simulink model "part_3_2"  (R2025a)
settings: Solver=FixedStepAuto  StartTime=0.0  StopTime=400  FixedStep=0.0005  RelTol=1e-3
values from neighbouring files (symbols this model uses):
  kts_to_ms = 0.5144444444    [constants.m]
  q0 = 0    [part_3_2_params.m]
  theta_f_0 = atan2(-D0,p.W)    [part_3_2_params.m]
  u0 = V0 * cos(theta_f_0)    [part_3_2_params.m]
  w0 = V0 * sin(theta_f_0)    [part_3_2_params.m]
undefined symbols (not defined in the file or in its folder): theta_0_trim
libraries: slpidlib x3, simulink x1
settings Model: Creator=niels  LastModifiedBy=niels

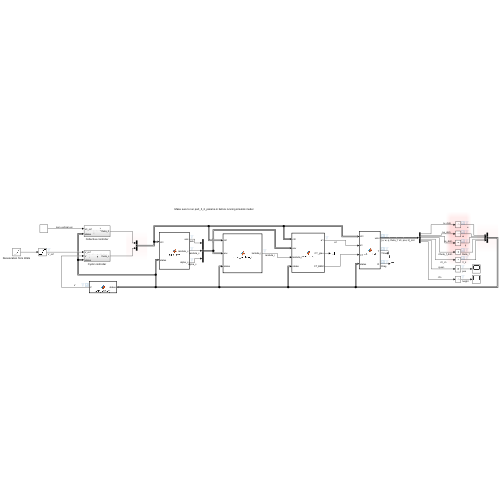
[thumbnail: Simulink's stored preview of the top-level diagram]
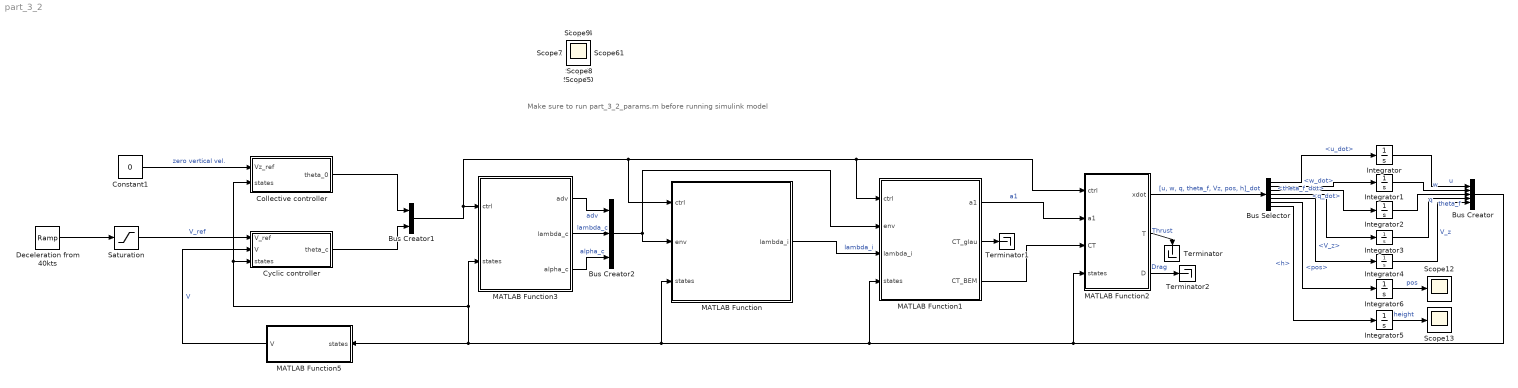
== system part_3_2 ==
  note: Make sure to run part_3_2_params.m before running simulink model
  Bus Creator : BusCreator  Inputs=5  OutDataTypeStr=Bus: slBus1
  Bus Creator1 : BusCreator  Inputs=2  OutDataTypeStr=Bus: slBus2
  Bus Creator2 : BusCreator  Inputs=3
  Bus Selector : BusSelector  OutputSignals=u_dot,w_dot,q_dot,theta_f_dot,V_z,pos,h
  Collective controller : Subsystem
  Constant1 : Constant  Value=0
  Cyclic controller : Subsystem
  Deceleration from 40kts : simulink/Sources/Ramp  slope=-1 * kts_to_ms  start=5  InitialOutput=40 * kts_to_ms
  Integrator : Integrator  InitialCondition=u0
  Integrator1 : Integrator  InitialCondition=w0
  Integrator2 : Integrator  InitialCondition=q0
  Integrator3 : Integrator  InitialCondition=theta_f_0
  Integrator4 : Integrator
  Integrator5 : Integrator
  Integrator6 : Integrator
  MATLAB Function : MATLAB Function  TreatAsAtomicUnit=on
  MATLAB Function1 : MATLAB Function  TreatAsAtomicUnit=on
  MATLAB Function2 : MATLAB Function  TreatAsAtomicUnit=on
  MATLAB Function3 : MATLAB Function  TreatAsAtomicUnit=on
  MATLAB Function5 : MATLAB Function  TreatAsAtomicUnit=on
  Saturation : Saturate  UpperLimit=40 * kts_to_ms  LowerLimit=0
  Scope{,1..13} (14 alike) : Scope
      Scope12 settings: ActiveDisplayYMinimum=-66.519454553298687  ActiveDisplayYMaximum=598.67509097968832  DataLoggingVariableName=ScopeData12
      Scope13 settings: ActiveDisplayYMinimum=-0.8759795141479535  ActiveDisplayYMaximum=0.71117795186084842  DataLoggingVariableName=ScopeData13
      Scope settings: ActiveDisplayYMinimum=-69.673258872485547  ActiveDisplayYMaximum=96.001341434570236
      Scope1 settings: ActiveDisplayYMinimum=-4.975868665333758  ActiveDisplayYMaximum=4.3203867980241615
      Scope10 settings: ActiveDisplayYMinimum=-1  ActiveDisplayYMaximum=1  DataLoggingVariableName=ScopeData10
      Scope11 settings: ActiveDisplayYMinimum=-0.16112339475038778  ActiveDisplayYMaximum=0.36190773098455026  DataLoggingVariableName=ScopeData11
      Scope2 settings: ActiveDisplayYMinimum=-0.593397020253839  ActiveDisplayYMaximum=52.786649391478015  DataLoggingVariableName=ScopeData2
      Scope3 settings: ActiveDisplayYMinimum=-78.6156985163187  ActiveDisplayYMaximum=71.050366553263416  DataLoggingVariableName=ScopeData3
      Scope4 settings: ActiveDisplayYMinimum=-4497.44134433289  ActiveDisplayYMaximum=2027.1404146909797  DataLoggingVariableName=ScopeData4
      Scope5 settings: ActiveDisplayYMinimum=-24353.236413473656  ActiveDisplayYMaximum=7406.41209327752  DataLoggingVariableName=ScopeData5
      Scope6 settings: DataLoggingVariableName=ScopeData6
      Scope7 settings: DataLoggingVariableName=ScopeData7
      Scope8 settings: ActiveDisplayYMinimum=-71153.912510590511  ActiveDisplayYMaximum=70611.962806822383  DataLoggingVariableName=ScopeData8
      Scope9 settings: ActiveDisplayYMinimum=-197167.0431723232  ActiveDisplayYMaximum=258208.12713879911  DataLoggingVariableName=ScopeData9
  Terminator : Terminator
  Terminator1 : Terminator
  Terminator2 : Terminator
  wires:
  MATLAB Function3/1(adv) -> Bus Creator2/1  "adv"
  MATLAB Function/1(lambda_i) -> MATLAB Function1/3(lambda_i)  "lambda_i"
  MATLAB Function1/1(a1) -> MATLAB Function2/2(a1)  "a1"
  MATLAB Function5/1(V) -> Cyclic controller/2(V)  "V"
  MATLAB Function1/3(CT_BEM) -> MATLAB Function2/3(CT)
  MATLAB Function3/2(lambda_c) -> Bus Creator2/2  "lambda_c"
  MATLAB Function3/3(alpha_c) -> Bus Creator2/3  "alpha_c"
  Bus Creator1/1 -> MATLAB Function2/1(ctrl), MATLAB Function1/1(ctrl), MATLAB Function/1(ctrl), MATLAB Function3/1(ctrl)
  MATLAB Function2/1(xdot) -> Bus Selector/1  "[u, w, q, theta_f, Vz, pos, h]_dot"
  Bus Selector/1 -> Integrator/1  "<u_dot>"
  Bus Selector/2 -> Integrator1/1  "<w_dot>"
  Integrator/1 -> Bus Creator/1  "u"
  Integrator1/1 -> Bus Creator/2  "w"
  Integrator2/1 -> Bus Creator/3  "q"
  Integrator3/1 -> Bus Creator/4  "theta_f"
  Bus Selector/3 -> Integrator2/1  "<q_dot>"
  Bus Creator/1 -> MATLAB Function2/4(states), MATLAB Function1/4(states), MATLAB Function/3(states), Collective controller/2(states), Cyclic controller/3(states), MATLAB Function3/2(states), MATLAB Function5/1(states)
  MATLAB Function2/2(T) -> Terminator/1  "Thrust"
  MATLAB Function2/3(D) -> Terminator2/1  "Drag"
  Bus Creator2/1 -> MATLAB Function/2(env), MATLAB Function1/2(env)
  Collective controller/1(theta_0) -> Bus Creator1/1
  Cyclic controller/1(theta_c) -> Bus Creator1/2
  Bus Selector/4 -> Integrator3/1  "<theta_f_dot>"
  Constant1/1 -> Collective controller/1(Vz_ref)  "zero vertical vel."
  Bus Selector/5 -> Integrator4/1  "<V_z>"
  Integrator4/1 -> Bus Creator/5  "V_z"
  Saturation/1 -> Cyclic controller/1(V_ref)  "V_ref"
  Deceleration from 40kts/1 -> Saturation/1
  Bus Selector/6 -> Integrator6/1  "<pos>"
  Bus Selector/7 -> Integrator5/1  "<h>"
  Integrator6/1 -> Scope12/1  "pos"
  Integrator5/1 -> Scope13/1  "height"
  MATLAB Function1/2(CT_glau) -> Terminator1/1

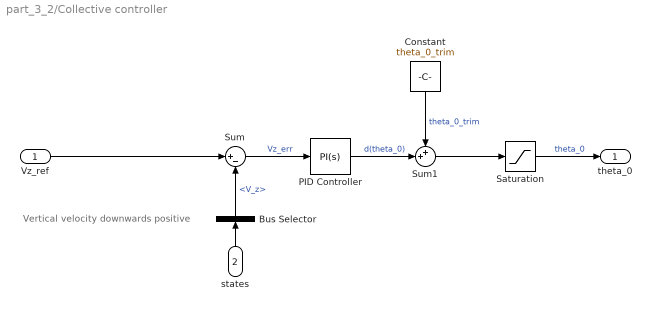
== system part_3_2/Collective controller ==
  note: Vertical velocity downwards positive
  Vz_ref : Inport
  states : Inport  Port=2
  Bus Selector : BusSelector  OutputSignals=V_z
  Constant : Constant  Value=theta_0_trim
  PID Controller : slpidlib/PID Controller  Controller=PI  Form=Parallel  TimeDomain=Continuous-time  UseExternalTs=off  SampleTime=-1  IntegratorMethod=Forward Euler  FilterMethod=Forward Euler  ControllerParametersSource=internal  P=0.356905218737675  I=3.63280538861423  UseKiTs=off  D=0  UseExternalDerivativeSource=off  N=100  UseFilter=on  TunerSelectOption=Transfer Function Based (PID Tuner App)  InitialConditionSource=internal  InitialConditionForIntegrator=0  InitialConditionForFilter=0  DifferentiatorICPrevScaledInput=0  ExternalReset=none  TrackingMode=off  Kt=1  LimitOutput=on  SatLimitsSource=internal  UpperSaturationLimit=inf  LowerSaturationLimit=-inf  LinearizeAsGain=on  AntiWindupMode=back-calculation  Kb=1/1.7722615314585  LimitIntegrator=off  UpperIntegratorSaturationLimit=inf  LowerIntegratorSaturationLimit=-inf  POutMin=[]  POutMax=[]  IOutMin=[]  IOutMax=[]  DOutMin=[]  DOutMax=[]  NOutMin=[]  NOutMax=[]  SumOutMin=[]  SumOutMax=[]  SaturationOutMin=[]  SaturationOutMax=[]  PParamMin=[]  PParamMax=[]  IParamMin=[]  IParamMax=[]  DParamMin=[]  DParamMax=[]  NParamMin=[]  NParamMax=[]  KbParamMin=[]  KbParamMax=[]  KtParamMin=[]  KtParamMax=[]  KbOutMin=[]  KbOutMax=[]  KtOutMin=[]  KtOutMax=[]  IntegratorOutMin=[]  IntegratorOutMax=[]  FilterOutMin=[]  FilterOutMax=[]  SumI1OutMin=[]  SumI1OutMax=[]  SumI2OutMin=[]  SumI2OutMax=[]  SumI3OutMin=[]  SumI3OutMax=[]  SumI4OutMin=[]  SumI4OutMax=[]  SumDOutMin=[]  SumDOutMax=[]  DifferentiatorOutMin=[]  DifferentiatorOutMax=[]  FilterDiffOutCoefMin=[]  FilterDiffOutCoefMax=[]  ReciprocalOutMin=[]  ReciprocalOutMax=[]  SumDenOutMin=[]  SumDenOutMax=[]  SumNumOutMin=[]  SumNumOutMax=[]  DivideOutMin=[]  DivideOutMax=[]  UdiffTsProdOutMin=[]  UdiffTsProdOutMax=[]  NTsProdOutMin=[]  NTsProdOutMax=[]  UintegralTsProdOutMin=[]  UintegralTsProdOutMax=[]  UngainTsProdOutMin=[]  UngainTsProdOutMax=[]  ClampingZeroOutDataTypeStr=Inherit: Inherit via back propagation  ClampingZeroOutMin=[]  ClampingZeroOutMax=[]  FilterDenConstantOutDataTypeStr=Inherit: Inherit via back propagation  FilterDenConstantOutMin=[]  FilterDenConstantOutMax=[]  PCopyOutDataTypeStr=Inherit: Inherit via back propagation  PCopyOutMin=[]  PCopyOutMax=[]  NCopyOutDataTypeStr=Inherit: Inherit via back propagation  NCopyOutMin=[]  NCopyOutMax=[]  IntegratorContinuousStateAttributes=''  IntegratorStateMustResolveToSignalObject=off  IntegratorRTWStateStorageClass=Auto  FilterContinuousStateAttributes=''  FilterStateMustResolveToSignalObject=off  FilterRTWStateStorageClass=Auto  ParallelPVariant=InternalParameters  IdealPVariant=Disabled  IVariant=InternalParameters  DVariant=Disabled  IntegratorVariant=Continuous  SatVariant=Enabled  AWVariant=BackCalculation  PCopyVariant=Disabled  TRVariant=Disabled  FdbkBlocksVariant=Forward  IdealPFdbkVariant=Disabled  SatFdbkVariant=Disabled  DerivativeFilterVariant=Disabled  NVariant=Disabled  NCopyVariant=Disabled_SignalSpec  FilterICVariant=Disabled  IntegratorICVariant=InternalICs  ExternalResetVariant=Disabled  TRSumVariant=Passthrough  SumFdbkVariant=Disabled  SumVariant=Sum_PI  TsampFilterVariant=InternalTs  TsampNgainVariant=Passthrough  TsampIntegralVariant=Disabled_SignalSpec  ExternalSaturationOutDataTypeStr=Inherit: Same as second input  DerivativeSourceVariant=Disabled  PreIntVariant=InternalPreInt
  Saturation : Saturate  UpperLimit=22.7*pi/180  LowerLimit=4*pi/180  LinearizeAsGain=off
  Sum : Sum  Inputs=|+-
  Sum1 : Sum  Inputs=++|
  theta_0 : Outport
  wires:
  Vz_ref/1 -> Sum/1
  Constant/1 -> Sum1/1  "theta_0_trim"
  Sum1/1 -> Saturation/1
  Sum/1 -> PID Controller/1  "Vz_err"
  PID Controller/1 -> Sum1/2  "d(theta_0)"
  Saturation/1 -> theta_0/1  "theta_0"
  states/1 -> Bus Selector/1
  Bus Selector/1 -> Sum/2  "<V_z>"

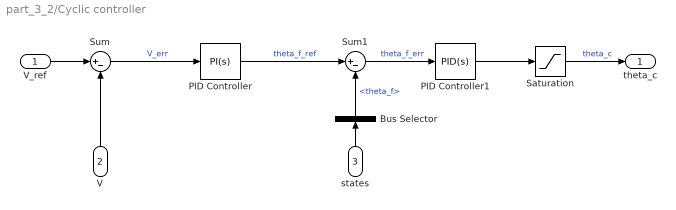
== system part_3_2/Cyclic controller ==
  V_ref : Inport
  V : Inport  Port=2
  states : Inport  Port=3
  Bus Selector : BusSelector  OutputSignals=theta_f
  PID Controller : slpidlib/PID Controller  Controller=PI  Form=Parallel  TimeDomain=Continuous-time  UseExternalTs=off  SampleTime=-1  IntegratorMethod=Forward Euler  FilterMethod=Forward Euler  ControllerParametersSource=internal  P=-0.0818787795811215  I=-0.000899384749307426  UseKiTs=off  D=0  UseExternalDerivativeSource=off  N=100  UseFilter=on  TunerSelectOption=Transfer Function Based (PID Tuner App)  InitialConditionSource=internal  InitialConditionForIntegrator=0  InitialConditionForFilter=0  DifferentiatorICPrevScaledInput=0  ExternalReset=none  TrackingMode=off  Kt=1  LimitOutput=off  SatLimitsSource=internal  UpperSaturationLimit=inf  LowerSaturationLimit=-inf  LinearizeAsGain=on  AntiWindupMode=none  Kb=1  LimitIntegrator=off  UpperIntegratorSaturationLimit=inf  LowerIntegratorSaturationLimit=-inf  POutMin=[]  POutMax=[]  IOutMin=[]  IOutMax=[]  DOutMin=[]  DOutMax=[]  NOutMin=[]  NOutMax=[]  SumOutMin=[]  SumOutMax=[]  SaturationOutMin=[]  SaturationOutMax=[]  PParamMin=[]  PParamMax=[]  IParamMin=[]  IParamMax=[]  DParamMin=[]  DParamMax=[]  NParamMin=[]  NParamMax=[]  KbParamMin=[]  KbParamMax=[]  KtParamMin=[]  KtParamMax=[]  KbOutMin=[]  KbOutMax=[]  KtOutMin=[]  KtOutMax=[]  IntegratorOutMin=[]  IntegratorOutMax=[]  FilterOutMin=[]  FilterOutMax=[]  SumI1OutMin=[]  SumI1OutMax=[]  SumI2OutMin=[]  SumI2OutMax=[]  SumI3OutMin=[]  SumI3OutMax=[]  SumI4OutMin=[]  SumI4OutMax=[]  SumDOutMin=[]  SumDOutMax=[]  DifferentiatorOutMin=[]  DifferentiatorOutMax=[]  FilterDiffOutCoefMin=[]  FilterDiffOutCoefMax=[]  ReciprocalOutMin=[]  ReciprocalOutMax=[]  SumDenOutMin=[]  SumDenOutMax=[]  SumNumOutMin=[]  SumNumOutMax=[]  DivideOutMin=[]  DivideOutMax=[]  UdiffTsProdOutMin=[]  UdiffTsProdOutMax=[]  NTsProdOutMin=[]  NTsProdOutMax=[]  UintegralTsProdOutMin=[]  UintegralTsProdOutMax=[]  UngainTsProdOutMin=[]  UngainTsProdOutMax=[]  ClampingZeroOutDataTypeStr=Inherit: Inherit via back propagation  ClampingZeroOutMin=[]  ClampingZeroOutMax=[]  FilterDenConstantOutDataTypeStr=Inherit: Inherit via back propagation  FilterDenConstantOutMin=[]  FilterDenConstantOutMax=[]  PCopyOutDataTypeStr=Inherit: Inherit via back propagation  PCopyOutMin=[]  PCopyOutMax=[]  NCopyOutDataTypeStr=Inherit: Inherit via back propagation  NCopyOutMin=[]  NCopyOutMax=[]  IntegratorContinuousStateAttributes=''  IntegratorStateMustResolveToSignalObject=off  IntegratorRTWStateStorageClass=Auto  FilterContinuousStateAttributes=''  FilterStateMustResolveToSignalObject=off  FilterRTWStateStorageClass=Auto  ParallelPVariant=InternalParameters  IdealPVariant=Disabled  IVariant=InternalParameters  DVariant=Disabled  IntegratorVariant=Continuous  SatVariant=Disabled  AWVariant=Passthrough  PCopyVariant=Disabled  TRVariant=Disabled  FdbkBlocksVariant=Forward  IdealPFdbkVariant=Disabled  SatFdbkVariant=Disabled  DerivativeFilterVariant=Disabled  NVariant=Disabled  NCopyVariant=Disabled_SignalSpec  FilterICVariant=Disabled  IntegratorICVariant=InternalICs  ExternalResetVariant=Disabled  TRSumVariant=Passthrough  SumFdbkVariant=Disabled  SumVariant=Sum_PI  TsampFilterVariant=InternalTs  TsampNgainVariant=Passthrough  TsampIntegralVariant=Disabled_SignalSpec  ExternalSaturationOutDataTypeStr=Inherit: Same as second input  DerivativeSourceVariant=Disabled  PreIntVariant=InternalPreInt
  PID Controller1 : slpidlib/PID Controller  Controller=PID  Form=Parallel  TimeDomain=Continuous-time  UseExternalTs=off  SampleTime=-1  IntegratorMethod=Forward Euler  FilterMethod=Forward Euler  ControllerParametersSource=internal  P=-74.2488008539596  I=-94.6679783127372  UseKiTs=off  D=-14.3024383116871  UseExternalDerivativeSource=off  N=147.428825111733  UseFilter=on  TunerSelectOption=Transfer Function Based (PID Tuner App)  InitialConditionSource=internal  InitialConditionForIntegrator=0  InitialConditionForFilter=0  DifferentiatorICPrevScaledInput=0  ExternalReset=none  TrackingMode=off  Kt=1  LimitOutput=off  SatLimitsSource=internal  UpperSaturationLimit=inf  LowerSaturationLimit=-inf  LinearizeAsGain=on  AntiWindupMode=back-calculation  Kb=1/22.8221920607983  LimitIntegrator=off  UpperIntegratorSaturationLimit=inf  LowerIntegratorSaturationLimit=-inf  POutMin=[]  POutMax=[]  IOutMin=[]  IOutMax=[]  DOutMin=[]  DOutMax=[]  NOutMin=[]  NOutMax=[]  SumOutMin=[]  SumOutMax=[]  SaturationOutMin=[]  SaturationOutMax=[]  PParamMin=[]  PParamMax=[]  IParamMin=[]  IParamMax=[]  DParamMin=[]  DParamMax=[]  NParamMin=[]  NParamMax=[]  KbParamMin=[]  KbParamMax=[]  KtParamMin=[]  KtParamMax=[]  KbOutMin=[]  KbOutMax=[]  KtOutMin=[]  KtOutMax=[]  IntegratorOutMin=[]  IntegratorOutMax=[]  FilterOutMin=[]  FilterOutMax=[]  SumI1OutMin=[]  SumI1OutMax=[]  SumI2OutMin=[]  SumI2OutMax=[]  SumI3OutMin=[]  SumI3OutMax=[]  SumI4OutMin=[]  SumI4OutMax=[]  SumDOutMin=[]  SumDOutMax=[]  DifferentiatorOutMin=[]  DifferentiatorOutMax=[]  FilterDiffOutCoefMin=[]  FilterDiffOutCoefMax=[]  ReciprocalOutMin=[]  ReciprocalOutMax=[]  SumDenOutMin=[]  SumDenOutMax=[]  SumNumOutMin=[]  SumNumOutMax=[]  DivideOutMin=[]  DivideOutMax=[]  UdiffTsProdOutMin=[]  UdiffTsProdOutMax=[]  NTsProdOutMin=[]  NTsProdOutMax=[]  UintegralTsProdOutMin=[]  UintegralTsProdOutMax=[]  UngainTsProdOutMin=[]  UngainTsProdOutMax=[]  ClampingZeroOutDataTypeStr=Inherit: Inherit via back propagation  ClampingZeroOutMin=[]  ClampingZeroOutMax=[]  FilterDenConstantOutDataTypeStr=Inherit: Inherit via back propagation  FilterDenConstantOutMin=[]  FilterDenConstantOutMax=[]  PCopyOutDataTypeStr=Inherit: Inherit via back propagation  PCopyOutMin=[]  PCopyOutMax=[]  NCopyOutDataTypeStr=Inherit: Inherit via back propagation  NCopyOutMin=[]  NCopyOutMax=[]  IntegratorContinuousStateAttributes=''  IntegratorStateMustResolveToSignalObject=off  IntegratorRTWStateStorageClass=Auto  FilterContinuousStateAttributes=''  FilterStateMustResolveToSignalObject=off  FilterRTWStateStorageClass=Auto  ParallelPVariant=InternalParameters  IdealPVariant=Disabled  IVariant=InternalParameters  DVariant=InternalParameters  IntegratorVariant=Continuous  SatVariant=Disabled  AWVariant=Passthrough  PCopyVariant=Disabled  TRVariant=Disabled  FdbkBlocksVariant=Forward  IdealPFdbkVariant=Disabled  SatFdbkVariant=Disabled  DerivativeFilterVariant=ContFilter  NVariant=InternalParameters  NCopyVariant=Disabled  FilterICVariant=InternalICsFilter  IntegratorICVariant=InternalICs  ExternalResetVariant=Disabled  TRSumVariant=Passthrough  SumFdbkVariant=Disabled  SumVariant=Sum_PID  TsampFilterVariant=InternalTs  TsampNgainVariant=Passthrough  TsampIntegralVariant=Disabled_SignalSpec  ExternalSaturationOutDataTypeStr=Inherit: Same as second input  DerivativeSourceVariant=ErrorSignal  PreIntVariant=InternalPreInt
  Saturation : Saturate  UpperLimit=19.25*pi/180  LowerLimit=-14.75*pi/180
  Sum : Sum  Inputs=|+-
  Sum1 : Sum  Inputs=|+-
  theta_c : Outport
  wires:
  V_ref/1 -> Sum/1
  V/1 -> Sum/2
  Sum/1 -> PID Controller/1  "V_err"
  Sum1/1 -> PID Controller1/1  "theta_f_err"
  PID Controller1/1 -> Saturation/1
  Saturation/1 -> theta_c/1  "theta_c"
  PID Controller/1 -> Sum1/1  "theta_f_ref"
  states/1 -> Bus Selector/1
  Bus Selector/1 -> Sum1/2  "<theta_f>"

== matlab function part_3_2/MATLAB Function1 ==
  data: ctrl input Bus: slBus2; env input Bus: slBus4; lambda_i input; a1 output; CT_glau output; states input Bus: slBus1; CT_BEM output; p parameter
function [a1, CT_glau, CT_BEM] = ...
            calc_aero(ctrl, env, lambda_i, states, p)

    theta_0 = ctrl.theta_0;
    q = states.q;
    adv = env.adv;
    lambda_c = env.lambda_c;
    alpha_c = env.alpha_c;
    
    % a1: longitudinal flapping angle
    num   = (8/3)*adv*theta_0 - 2*adv*(lambda_c + lambda_i) ...
                - (16/p.Lock)*(q/p.OmegaR);
    den = 1 - 0.5*adv^2;
    if abs(den) < 1e-8
        den = sign(den + eps) * 1e-8;
    end
    
    a1 = num / den;

    % CT_BEM: Blade Element Momentum thrust coefficient
    CT_BEM = p.cl_alpha * (1/4) * (p.sigma) * ((2/3)*theta_0* ...
                (1 + (3/2)*adv^2) - (lambda_c + lambda_i));

    % CT_glau: Glauert thrust coefficient
    Vc_norm = adv * cos(alpha_c - a1);
    Vs_norm = adv * sin(alpha_c - a1);

    CT_glau = 2 * lambda_i * sqrt( Vc_norm^2 + (Vs_norm + lambda_i)^2 );

end

== matlab function part_3_2/MATLAB Function ==
  data: ctrl input Bus: slBus2; env input Bus: slBus4; lambda_i output; states input Bus: slBus1; p parameter
function lambda_i  = ...
            solve_lambda_i(ctrl, env, states, p)
% Solves for lambda_i such that F(lambda_i) = C_TBEM - C_TGlau = 0
%
% Inputs:
%   adv      - advance ratio [-]
%   theta_0  - collective pitch [rad]
%   lambda_c - climb inflow ratio
%   q        - some loading parameter
%   alpha_c  - shaft/disc tilt angle [rad]
%   p        - data struct
    theta_0 = ctrl.theta_0;
    q = states.q;
    adv = env.adv;
    lambda_c = env.lambda_c;
    alpha_c = env.alpha_c;

    % Define the residual function F(lambda_i) = C_TBEM - C_TGlau
    F = @(lambda_i) residual(lambda_i, adv, theta_0, lambda_c, q, ...
                                alpha_c, p);

    % Initial guess for lambda_i
    lambda_i0 = 0.05;

    % Solve using fzero
    lambda_i = fzero(F, lambda_i0);

    fprintf('Converged: lambda_i = %.6f\n', lambda_i);
end

function F = residual(lambda_i, adv, theta_0, lambda_c, q, alpha_c, p)

    % a1: longitudinal flapping angle
    num   = (8/3)*adv*theta_0 - 2*adv*(lambda_c + lambda_i) ...
                - (16/p.Lock)*(q/p.OmegaR);
    den = 1 - 0.5*adv^2;
    if abs(den) < 1e-8
        den = sign(den + eps) * 1e-8;
    end
    
    a1 = num / den;

    % CT_BEM: Blade Element Momentum thrust coefficient
    CT_BEM = p.cl_alpha * (1/4) * (p.sigma) * ((2/3)*theta_0* ...
                (1 + (3/2)*adv^2) - (lambda_c + lambda_i));

    % CT_glau: Glauert thrust coefficient
    Vc_norm = adv * cos(alpha_c - a1);
    Vs_norm = adv * sin(alpha_c - a1);

    CT_glau = 2 * lambda_i * sqrt( Vc_norm^2 + (Vs_norm + lambda_i)^2 );

    % Residual
    F = CT_BEM - CT_glau;
end

== matlab function part_3_2/MATLAB Function2 ==
  data: ctrl input Bus: slBus2; a1 input; CT input; states input Bus: slBus1; xdot output Bus: slBus3; p parameter; T output; D output
function [xdot, T, D] = calc_EOM(ctrl, a1, CT, states, p)
    % unpack states and controls
    u = states.u; w = states.w; q = states.q; theta_f = states.theta_f; 
    V_z = states.V_z;
    theta_c = ctrl.theta_c;
    
    V = sqrt(u^2 + w^2);
    if V < 1e-8
        V = sign(V + eps) * 1e-8;
    end

    % Calculate thrust and drag
    T = CT * p.rho * p.OmegaR^2 * p.A;
    D = p.A_eq * 1/2 * p.rho * V^2;

    % Calculate state derivatives
    if V < 0.1
        xdot.u_dot = -p.g * sin(theta_f) + T/p.m * sin(theta_c - a1);
        xdot.w_dot = p.g * cos(theta_f) - T/p.m * cos(theta_c - a1);
    else
        xdot.u_dot = -p.g * sin(theta_f) - D/p.m * u/V ...
                    + T/p.m * sin(theta_c - a1) - q*w;
        xdot.w_dot = p.g * cos(theta_f) - D/p.m * w/V ...
                    - T/p.m * cos(theta_c - a1) + q*u;
    end
    
    xdot.q_dot = -T/p.Iy * p.h * sin(theta_c - a1);
    xdot.theta_f_dot = q;
    xdot.V_z = - xdot.w_dot * cos(theta_f) + w * sin(theta_f) * q ...
                + xdot.u_dot * sin(theta_f) + u * cos(theta_f) * q;
    xdot.pos = u * cos(theta_f) - w * sin(theta_f);
    xdot.h = V_z;
end

== matlab function part_3_2/MATLAB Function3 ==
  data: ctrl input Bus: slBus2; adv output; lambda_c output; alpha_c output; states input Bus: slBus1; p parameter
function [adv, lambda_c, alpha_c] = calc_env(ctrl, states, p)
    % unpack states and controls
    u = states.u; w = states.w; q = states.q; theta_f = states.theta_f;
    theta_0 = ctrl.theta_0; theta_c = ctrl.theta_c;
    
    V = sqrt(u^2 + w^2);
    alpha_c = theta_c - atan2(w, u);
    adv = V / p.OmegaR * cos(alpha_c);
    lambda_c = V / p.OmegaR * sin(alpha_c);
end

== matlab function part_3_2/MATLAB Function5 ==
  data: states input; V output
function V = calc_velocity(states)
    u = states.u ; w = states.w;
    V = sign(u) * sqrt(u^2 + w^2);
end
